simulink model "shem5_1"  (R2023a)
settings: Solver=VariableStepAuto  StartTime=0.0  StopTime=10.0  RelTol=1e-3
settings Model: Creator=fynjy  LastModifiedBy=fynjy

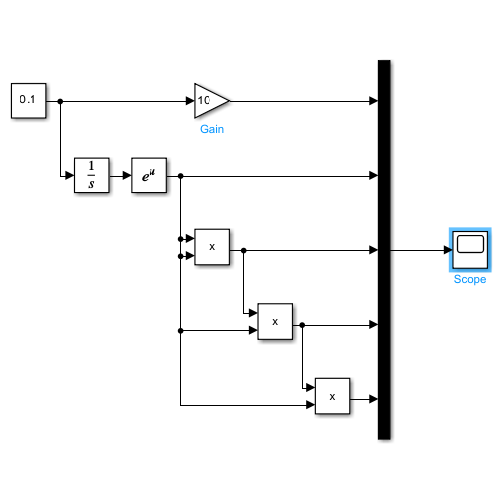
[thumbnail: Simulink's stored preview of the top-level diagram]
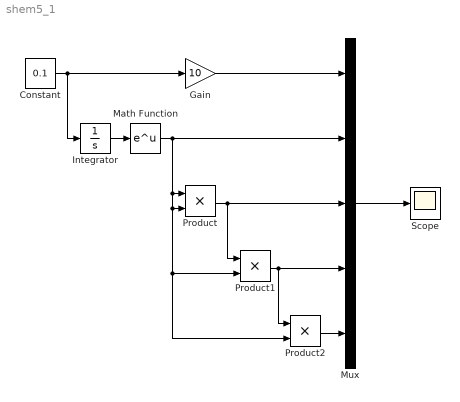
== system shem5_1 ==
  Constant : Constant  Value=0.1
  Gain : Gain  Gain=10
  Integrator : Integrator
  Math Function : Math
  Mux : Mux  Inputs=5
  Product : Product
  Product1 : Product
  Product2 : Product
  Scope : Scope
  wires:
  Mux/1 -> Scope/1
  Product2/1 -> Mux/5
  Product1/1 -> Product2/1, Mux/4
  Product/1 -> Product1/1, Mux/3
  Math Function/1 -> Product2/2, Product1/2, Product/2, Product/1, Mux/2
  Integrator/1 -> Math Function/1
  Constant/1 -> Integrator/1, Gain/1
  Gain/1 -> Mux/1
